simulink model "Counter"  (R2021a)
settings: Solver=VariableStepAuto  StartTime=0.0  StopTime=10.0  RelTol=1e-3
settings Model: Creator=Osman  LastModifiedBy=Osman

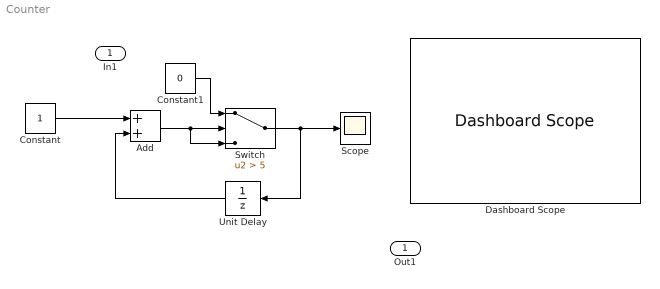
== system Counter ==
  In1 : Inport
  Add : Sum
  Constant : Constant  OutDataTypeStr=int32
  Constant1 : Constant  Value=0  OutDataTypeStr=int32
  Dashboard Scope : DashboardScope
  Scope : Scope
  Switch : Switch  Criteria=u2 > Threshold  Threshold=5  OutDataTypeStr=int32
  Unit Delay : UnitDelay  InitialCondition=-1  SampleTime=-1  HasFrameUpgradeWarning=on
  Out1 : Outport
  wires:
  Constant/1 -> Add/1
  Add/1 -> Switch/3, Switch/2
  Switch/1 -> Unit Delay/1, Scope/1
  Unit Delay/1 -> Add/2
  Constant1/1 -> Switch/1
